simulink model "EulerEqs"  (R2020b)
settings: Solver=VariableStepAuto  StartTime=0.0  StopTime=200  RelTol=1E-6  AbsTol=1E-4
values from neighbouring files (symbols this model uses):
  sim_constants = struct    [constants.m]
libraries: vrlib x1
settings Model: Creator=newpo  LastModifiedBy=newpo

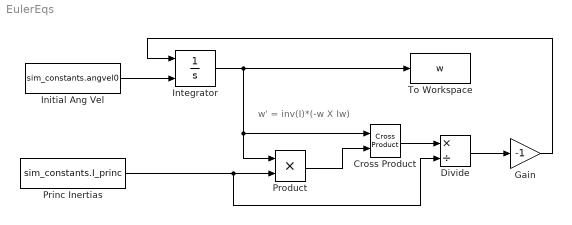
== system EulerEqs ==
  note: w' = inv(I)*(-w X Iw)
  Cross Product : vrlib/Utilities/Cross Product
  Divide : Product  Inputs=*/
  Gain : Gain  Gain=-1
  Initial Ang Vel : Constant  Value=sim_constants.angvel0
  Integrator : Integrator  InitialConditionSource=external
  Princ Inertias : Constant  Value=sim_constants.I_princ
  Product : Product
  To Workspace : ToWorkspace  VariableName=w  SampleTime=-1
  wires:
  Integrator/1 -> Cross Product/1, Product/1, To Workspace/1
  Gain/1 -> Integrator/1
  Cross Product/1 -> Divide/1
  Princ Inertias/1 -> Product/2, Divide/2
  Product/1 -> Cross Product/2
  Divide/1 -> Gain/1
  Initial Ang Vel/1 -> Integrator/2
